simulink model "cantx_0x191"  (R2022a)
settings: configuration reference "SLDD_CFG" (kept outside this file)
values from neighbouring files (symbols this model uses):
  PLCANI_APCNTL_SET_INF_2X = 0    [cantx_0x191.sldd]
  PLCANI_APCNTL_SET_INF_4X = 1    [cantx_0x191.sldd]
  PLCANI_APCNTL_SET_INF_8X = 2    [cantx_0x191.sldd]
  PLCANI_APCNTL_SET_INF_INIT = 99    [cantx_0x191.sldd]
libraries: simulink x12
settings Model: DataDictionary=cantx_0x191.sldd  Creator=Castiel  LastModifiedBy=Castiel
settings ConfigSetRef: SourceName=SLDD_CFG

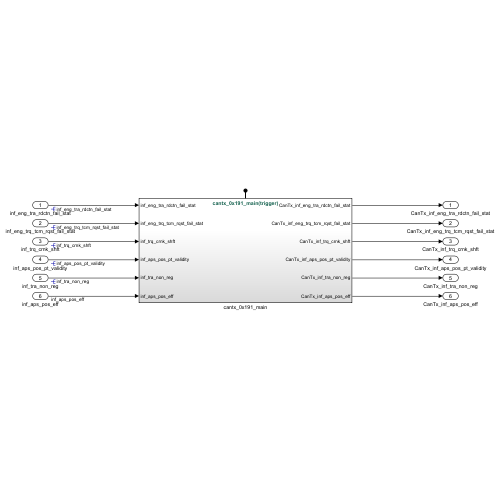
[thumbnail: Simulink's stored preview of the top-level diagram]
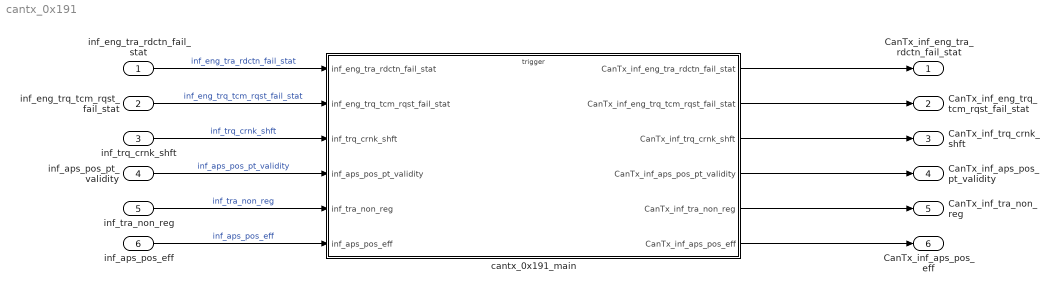
== system cantx_0x191 ==
  inf_eng_tra_rdctn_fail_stat : Inport
  inf_eng_trq_tcm_rqst_fail_stat : Inport  Port=2
  inf_trq_crnk_shft : Inport  Port=3
  inf_aps_pos_pt_validity : Inport  Port=4
  inf_tra_non_reg : Inport  Port=5
  inf_aps_pos_eff : Inport  Port=6
  cantx_0x191_main : Subsystem  TreatAsAtomicUnit=on
  CanTx_inf_eng_tra_rdctn_fail_stat : Outport  SignalName=CanTx_inf_eng_tra_rdctn_fail_stat
      settings: MustResolveToSignalObject=on
  CanTx_inf_eng_trq_tcm_rqst_fail_stat : Outport  Port=2  SignalName=CanTx_inf_eng_trq_tcm_rqst_fail_stat
      settings: MustResolveToSignalObject=on
  CanTx_inf_trq_crnk_shft : Outport  Port=3  SignalName=CanTx_inf_trq_crnk_shft
      settings: MustResolveToSignalObject=on
  CanTx_inf_aps_pos_pt_validity : Outport  Port=4  SignalName=CanTx_inf_aps_pos_pt_validity
      settings: MustResolveToSignalObject=on
  CanTx_inf_tra_non_reg : Outport  Port=5  SignalName=CanTx_inf_tra_non_reg
      settings: MustResolveToSignalObject=on
  CanTx_inf_aps_pos_eff : Outport  Port=6  SignalName=CanTx_inf_aps_pos_eff
      settings: MustResolveToSignalObject=on
  wires:
  inf_eng_tra_rdctn_fail_stat/1 -> cantx_0x191_main/1(inf_eng_tra_rdctn_fail_stat)  "inf_eng_tra_rdctn_fail_stat"
  inf_eng_trq_tcm_rqst_fail_stat/1 -> cantx_0x191_main/2(inf_eng_trq_tcm_rqst_fail_stat)  "inf_eng_trq_tcm_rqst_fail_stat"
  inf_trq_crnk_shft/1 -> cantx_0x191_main/3(inf_trq_crnk_shft)  "inf_trq_crnk_shft"
  inf_aps_pos_pt_validity/1 -> cantx_0x191_main/4(inf_aps_pos_pt_validity)  "inf_aps_pos_pt_validity"
  inf_tra_non_reg/1 -> cantx_0x191_main/5(inf_tra_non_reg)  "inf_tra_non_reg"
  inf_aps_pos_eff/1 -> cantx_0x191_main/6(inf_aps_pos_eff)  "inf_aps_pos_eff"
  cantx_0x191_main/1(CanTx_inf_eng_tra_rdctn_fail_stat) -> CanTx_inf_eng_tra_rdctn_fail_stat/1
  cantx_0x191_main/2(CanTx_inf_eng_trq_tcm_rqst_fail_stat) -> CanTx_inf_eng_trq_tcm_rqst_fail_stat/1
  cantx_0x191_main/3(CanTx_inf_trq_crnk_shft) -> CanTx_inf_trq_crnk_shft/1
  cantx_0x191_main/4(CanTx_inf_aps_pos_pt_validity) -> CanTx_inf_aps_pos_pt_validity/1
  cantx_0x191_main/5(CanTx_inf_tra_non_reg) -> CanTx_inf_tra_non_reg/1
  cantx_0x191_main/6(CanTx_inf_aps_pos_eff) -> CanTx_inf_aps_pos_eff/1

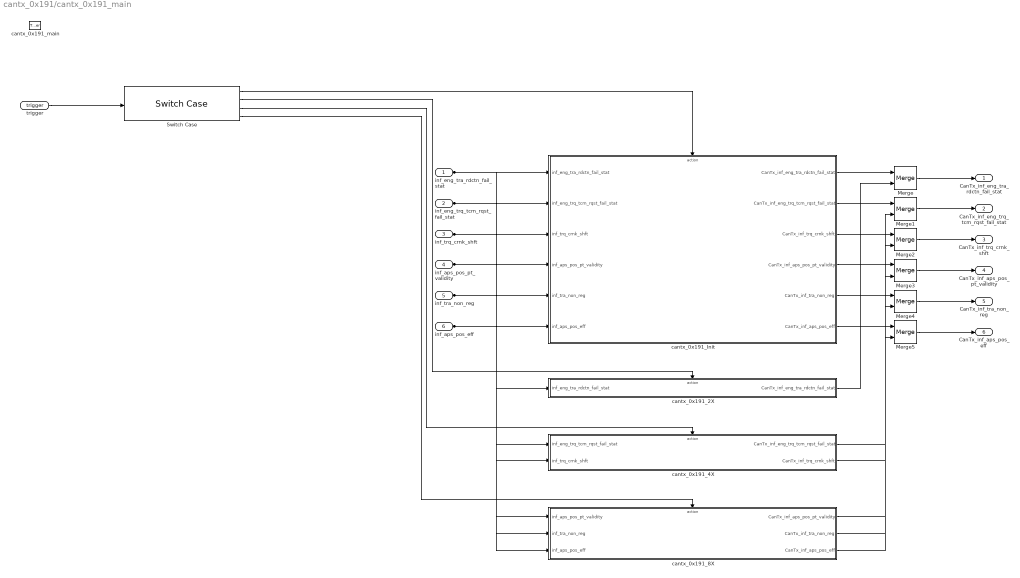
== system cantx_0x191/cantx_0x191_main ==
  inf_eng_tra_rdctn_fail_stat : Inport
  inf_eng_trq_tcm_rqst_fail_stat : Inport  Port=2
  inf_trq_crnk_shft : Inport  Port=3
  inf_aps_pos_pt_validity : Inport  Port=4
  inf_tra_non_reg : Inport  Port=5
  inf_aps_pos_eff : Inport  Port=6
  cantx_0x191_main : TriggerPort  TriggerType=function-call  IsSimulinkFunction=on  FunctionName=cantx_0x191_main  FunctionVisibility=scoped  VariantControl=(inherit)
  Merge{,1..5} (6 alike) : Merge
  Switch Case : SwitchCase  CaseConditions={PLCANI_APCNTL_SET_INF_TYPE.PLCANI_APCNTL_SET_INF_INIT,PLCANI_APCNTL_SET_INF_TYPE.PLCANI_APCNTL_SET_INF_2X,PLCANI_APCNTL_SET_INF_TYPE.PLCANI_APCNTL_SET_INF_4X,PLCANI_APCNTL_SET_INF_TYPE.PLCANI_APCNTL_SET_INF_8X}  ShowDefaultCase=off
  cantx_0x191_2X : Subsystem  TreatAsAtomicUnit=on
      settings: RTWFcnNameOpts=Use subsystem name
  cantx_0x191_4X : Subsystem  TreatAsAtomicUnit=on
      settings: RTWFcnNameOpts=Use subsystem name
  cantx_0x191_8X : Subsystem  TreatAsAtomicUnit=on
      settings: RTWFcnNameOpts=Use subsystem name
  cantx_0x191_Init : Subsystem  TreatAsAtomicUnit=on
      settings: RTWFcnNameOpts=Use subsystem name
  trigger : ArgIn  DisableCoverage=on  OutDataTypeStr=Enum: PLCANI_APCNTL_SET_INF_TYPE  ArgumentName=trigger
  CanTx_inf_eng_tra_rdctn_fail_stat : Outport
  CanTx_inf_eng_trq_tcm_rqst_fail_stat : Outport  Port=2
  CanTx_inf_trq_crnk_shft : Outport  Port=3
  CanTx_inf_aps_pos_pt_validity : Outport  Port=4
  CanTx_inf_tra_non_reg : Outport  Port=5
  CanTx_inf_aps_pos_eff : Outport  Port=6
  wires:
  trigger/1 -> Switch Case/1
  Switch Case/1 -> cantx_0x191_Init/Action
  inf_eng_tra_rdctn_fail_stat/1 -> cantx_0x191_Init/1(inf_eng_tra_rdctn_fail_stat), cantx_0x191_2X/1(inf_eng_tra_rdctn_fail_stat)
  inf_eng_trq_tcm_rqst_fail_stat/1 -> cantx_0x191_Init/2(inf_eng_trq_tcm_rqst_fail_stat), cantx_0x191_4X/1(inf_eng_trq_tcm_rqst_fail_stat)
  inf_trq_crnk_shft/1 -> cantx_0x191_Init/3(inf_trq_crnk_shft), cantx_0x191_4X/2(inf_trq_crnk_shft)
  inf_aps_pos_pt_validity/1 -> cantx_0x191_Init/4(inf_aps_pos_pt_validity), cantx_0x191_8X/1(inf_aps_pos_pt_validity)
  inf_tra_non_reg/1 -> cantx_0x191_Init/5(inf_tra_non_reg), cantx_0x191_8X/2(inf_tra_non_reg)
  inf_aps_pos_eff/1 -> cantx_0x191_Init/6(inf_aps_pos_eff), cantx_0x191_8X/3(inf_aps_pos_eff)
  Switch Case/2 -> cantx_0x191_2X/Action
  cantx_0x191_Init/1(CanTx_inf_eng_tra_rdctn_fail_stat) -> Merge/1
  cantx_0x191_2X/1(CanTx_inf_eng_tra_rdctn_fail_stat) -> Merge/2
  Merge/1 -> CanTx_inf_eng_tra_rdctn_fail_stat/1
  Switch Case/3 -> cantx_0x191_4X/Action
  cantx_0x191_Init/2(CanTx_inf_eng_trq_tcm_rqst_fail_stat) -> Merge1/1
  cantx_0x191_4X/1(CanTx_inf_eng_trq_tcm_rqst_fail_stat) -> Merge1/2
  Merge1/1 -> CanTx_inf_eng_trq_tcm_rqst_fail_stat/1
  cantx_0x191_Init/3(CanTx_inf_trq_crnk_shft) -> Merge2/1
  cantx_0x191_4X/2(CanTx_inf_trq_crnk_shft) -> Merge2/2
  Merge2/1 -> CanTx_inf_trq_crnk_shft/1
  Switch Case/4 -> cantx_0x191_8X/Action
  cantx_0x191_Init/4(CanTx_inf_aps_pos_pt_validity) -> Merge3/1
  cantx_0x191_8X/1(CanTx_inf_aps_pos_pt_validity) -> Merge3/2
  Merge3/1 -> CanTx_inf_aps_pos_pt_validity/1
  cantx_0x191_Init/5(CanTx_inf_tra_non_reg) -> Merge4/1
  cantx_0x191_8X/2(CanTx_inf_tra_non_reg) -> Merge4/2
  Merge4/1 -> CanTx_inf_tra_non_reg/1
  cantx_0x191_Init/6(CanTx_inf_aps_pos_eff) -> Merge5/1
  cantx_0x191_8X/3(CanTx_inf_aps_pos_eff) -> Merge5/2
  Merge5/1 -> CanTx_inf_aps_pos_eff/1

== system cantx_0x191/cantx_0x191_main/cantx_0x191_2X ==
  inf_eng_tra_rdctn_fail_stat : Inport
  Action Port : ActionPort  ActionPortLabel=case [ PLCANI_APCNTL_SET_INF_2X ]:
  sig_inf_eng_tra_rdctn_fail_stat : Subsystem  TreatAsAtomicUnit=on
      settings: RTWFcnNameOpts=Use subsystem name
  CanTx_inf_eng_tra_rdctn_fail_stat : Outport
  wires:
  inf_eng_tra_rdctn_fail_stat/1 -> sig_inf_eng_tra_rdctn_fail_stat/1(inf_eng_tra_rdctn_fail_stat)
  sig_inf_eng_tra_rdctn_fail_stat/1(CanTx_inf_eng_tra_rdctn_fail_stat) -> CanTx_inf_eng_tra_rdctn_fail_stat/1

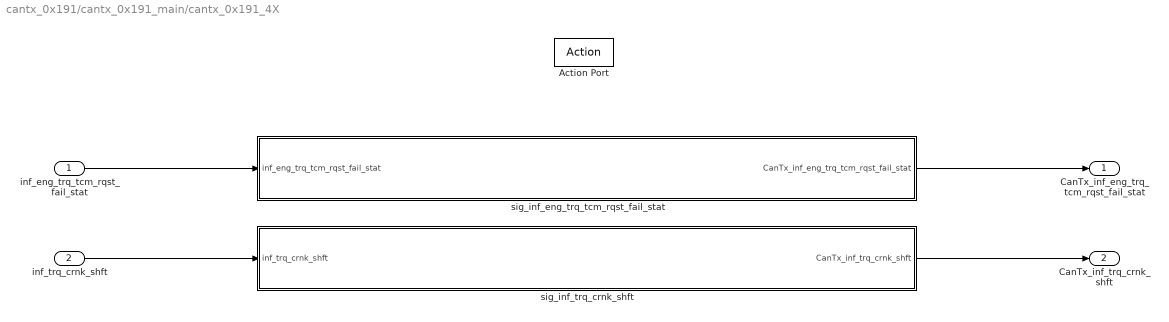
== system cantx_0x191/cantx_0x191_main/cantx_0x191_4X ==
  inf_eng_trq_tcm_rqst_fail_stat : Inport
  inf_trq_crnk_shft : Inport  Port=2
  Action Port : ActionPort  ActionPortLabel=case [ PLCANI_APCNTL_SET_INF_4X ]:
  sig_inf_eng_trq_tcm_rqst_fail_stat : Subsystem  TreatAsAtomicUnit=on
      settings: RTWFcnNameOpts=Use subsystem name
  sig_inf_trq_crnk_shft : Subsystem  TreatAsAtomicUnit=on
      settings: RTWFcnNameOpts=Use subsystem name
  CanTx_inf_eng_trq_tcm_rqst_fail_stat : Outport
  CanTx_inf_trq_crnk_shft : Outport  Port=2
  wires:
  inf_eng_trq_tcm_rqst_fail_stat/1 -> sig_inf_eng_trq_tcm_rqst_fail_stat/1(inf_eng_trq_tcm_rqst_fail_stat)
  sig_inf_eng_trq_tcm_rqst_fail_stat/1(CanTx_inf_eng_trq_tcm_rqst_fail_stat) -> CanTx_inf_eng_trq_tcm_rqst_fail_stat/1
  inf_trq_crnk_shft/1 -> sig_inf_trq_crnk_shft/1(inf_trq_crnk_shft)
  sig_inf_trq_crnk_shft/1(CanTx_inf_trq_crnk_shft) -> CanTx_inf_trq_crnk_shft/1

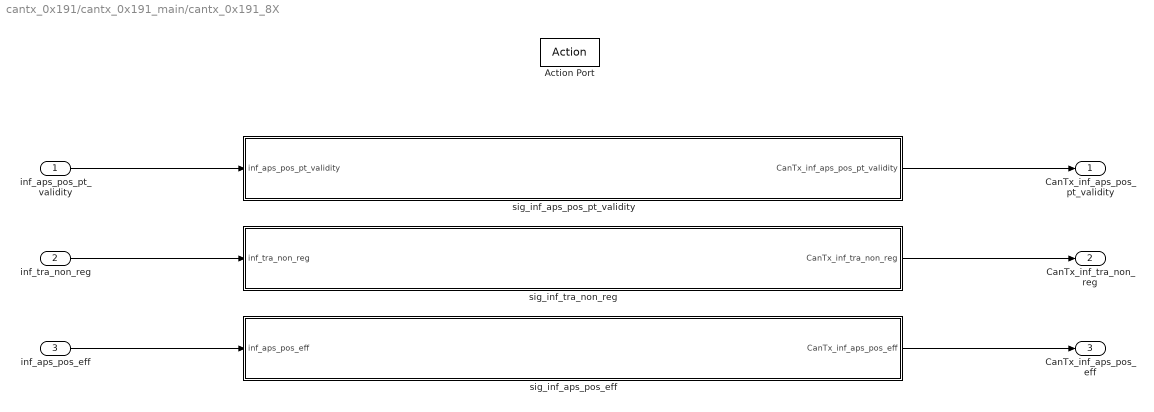
== system cantx_0x191/cantx_0x191_main/cantx_0x191_8X ==
  inf_aps_pos_pt_validity : Inport
  inf_tra_non_reg : Inport  Port=2
  inf_aps_pos_eff : Inport  Port=3
  Action Port : ActionPort  ActionPortLabel=case [ PLCANI_APCNTL_SET_INF_8X ]:
  sig_inf_aps_pos_eff : Subsystem  TreatAsAtomicUnit=on
      settings: RTWFcnNameOpts=Use subsystem name
  sig_inf_aps_pos_pt_validity : Subsystem  TreatAsAtomicUnit=on
      settings: RTWFcnNameOpts=Use subsystem name
  sig_inf_tra_non_reg : Subsystem  TreatAsAtomicUnit=on
      settings: RTWFcnNameOpts=Use subsystem name
  CanTx_inf_aps_pos_pt_validity : Outport
  CanTx_inf_tra_non_reg : Outport  Port=2
  CanTx_inf_aps_pos_eff : Outport  Port=3
  wires:
  inf_aps_pos_pt_validity/1 -> sig_inf_aps_pos_pt_validity/1(inf_aps_pos_pt_validity)
  sig_inf_aps_pos_pt_validity/1(CanTx_inf_aps_pos_pt_validity) -> CanTx_inf_aps_pos_pt_validity/1
  inf_tra_non_reg/1 -> sig_inf_tra_non_reg/1(inf_tra_non_reg)
  sig_inf_tra_non_reg/1(CanTx_inf_tra_non_reg) -> CanTx_inf_tra_non_reg/1
  inf_aps_pos_eff/1 -> sig_inf_aps_pos_eff/1(inf_aps_pos_eff)
  sig_inf_aps_pos_eff/1(CanTx_inf_aps_pos_eff) -> CanTx_inf_aps_pos_eff/1

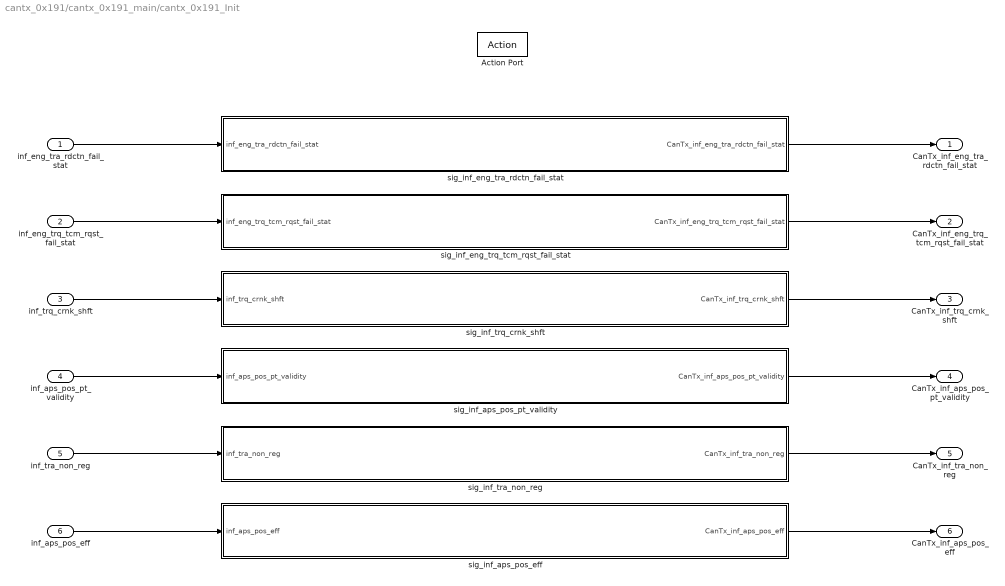
== system cantx_0x191/cantx_0x191_main/cantx_0x191_Init ==
  inf_eng_tra_rdctn_fail_stat : Inport
  inf_eng_trq_tcm_rqst_fail_stat : Inport  Port=2
  inf_trq_crnk_shft : Inport  Port=3
  inf_aps_pos_pt_validity : Inport  Port=4
  inf_tra_non_reg : Inport  Port=5
  inf_aps_pos_eff : Inport  Port=6
  Action Port : ActionPort  ActionPortLabel=case [ PLCANI_APCNTL_SET_INF_INIT ]:
  sig_inf_aps_pos_eff : Subsystem  TreatAsAtomicUnit=on
      settings: RTWFcnNameOpts=Use subsystem name
  sig_inf_aps_pos_pt_validity : Subsystem  TreatAsAtomicUnit=on
      settings: RTWFcnNameOpts=Use subsystem name
  sig_inf_eng_tra_rdctn_fail_stat : Subsystem  TreatAsAtomicUnit=on
      settings: RTWFcnNameOpts=Use subsystem name
  sig_inf_eng_trq_tcm_rqst_fail_stat : Subsystem  TreatAsAtomicUnit=on
      settings: RTWFcnNameOpts=Use subsystem name
  sig_inf_tra_non_reg : Subsystem  TreatAsAtomicUnit=on
      settings: RTWFcnNameOpts=Use subsystem name
  sig_inf_trq_crnk_shft : Subsystem  TreatAsAtomicUnit=on
      settings: RTWFcnNameOpts=Use subsystem name
  CanTx_inf_eng_tra_rdctn_fail_stat : Outport
  CanTx_inf_eng_trq_tcm_rqst_fail_stat : Outport  Port=2
  CanTx_inf_trq_crnk_shft : Outport  Port=3
  CanTx_inf_aps_pos_pt_validity : Outport  Port=4
  CanTx_inf_tra_non_reg : Outport  Port=5
  CanTx_inf_aps_pos_eff : Outport  Port=6
  wires:
  inf_eng_tra_rdctn_fail_stat/1 -> sig_inf_eng_tra_rdctn_fail_stat/1(inf_eng_tra_rdctn_fail_stat)
  sig_inf_eng_tra_rdctn_fail_stat/1(CanTx_inf_eng_tra_rdctn_fail_stat) -> CanTx_inf_eng_tra_rdctn_fail_stat/1
  inf_eng_trq_tcm_rqst_fail_stat/1 -> sig_inf_eng_trq_tcm_rqst_fail_stat/1(inf_eng_trq_tcm_rqst_fail_stat)
  sig_inf_eng_trq_tcm_rqst_fail_stat/1(CanTx_inf_eng_trq_tcm_rqst_fail_stat) -> CanTx_inf_eng_trq_tcm_rqst_fail_stat/1
  inf_trq_crnk_shft/1 -> sig_inf_trq_crnk_shft/1(inf_trq_crnk_shft)
  sig_inf_trq_crnk_shft/1(CanTx_inf_trq_crnk_shft) -> CanTx_inf_trq_crnk_shft/1
  inf_aps_pos_pt_validity/1 -> sig_inf_aps_pos_pt_validity/1(inf_aps_pos_pt_validity)
  sig_inf_aps_pos_pt_validity/1(CanTx_inf_aps_pos_pt_validity) -> CanTx_inf_aps_pos_pt_validity/1
  inf_tra_non_reg/1 -> sig_inf_tra_non_reg/1(inf_tra_non_reg)
  sig_inf_tra_non_reg/1(CanTx_inf_tra_non_reg) -> CanTx_inf_tra_non_reg/1
  inf_aps_pos_eff/1 -> sig_inf_aps_pos_eff/1(inf_aps_pos_eff)
  sig_inf_aps_pos_eff/1(CanTx_inf_aps_pos_eff) -> CanTx_inf_aps_pos_eff/1

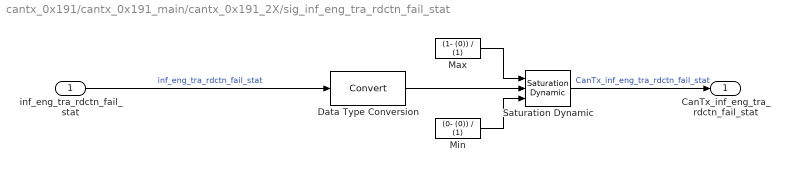
== system cantx_0x191/cantx_0x191_main/cantx_0x191_2X/sig_inf_eng_tra_rdctn_fail_stat ==
  inf_eng_tra_rdctn_fail_stat : Inport
  Data Type Conversion : DataTypeConversion  SaturateOnIntegerOverflow=off  RndMeth=Floor
  Max : Constant  Value=(1- (0)) / (1)  OutDataTypeStr=Inherit: Inherit via back propagation
  Min : Constant  Value=(0- (0)) / (1)  OutDataTypeStr=Inherit: Inherit via back propagation
  Saturation Dynamic : simulink/Discontinuities/Saturation Dynamic  OutMin=[]  OutMax=[]  OutDataTypeStr=Inherit: Same as second input  OutDataType=fixdt(1, 16)  OutScaling=2^-10  DoSatur=off
  CanTx_inf_eng_tra_rdctn_fail_stat : Outport
  wires:
  Saturation Dynamic/1 -> CanTx_inf_eng_tra_rdctn_fail_stat/1  "CanTx_inf_eng_tra_rdctn_fail_stat"
  Data Type Conversion/1 -> Saturation Dynamic/2
  inf_eng_tra_rdctn_fail_stat/1 -> Data Type Conversion/1  "inf_eng_tra_rdctn_fail_stat"
  Min/1 -> Saturation Dynamic/3
  Max/1 -> Saturation Dynamic/1

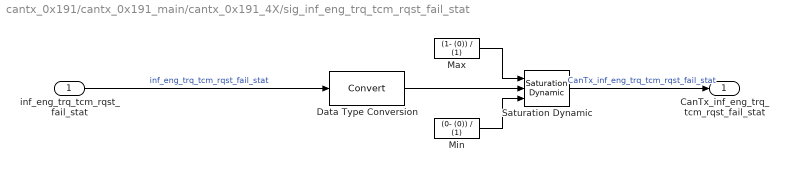
== system cantx_0x191/cantx_0x191_main/cantx_0x191_4X/sig_inf_eng_trq_tcm_rqst_fail_stat ==
  inf_eng_trq_tcm_rqst_fail_stat : Inport
  Data Type Conversion : DataTypeConversion  SaturateOnIntegerOverflow=off  RndMeth=Floor
  Max : Constant  Value=(1- (0)) / (1)  OutDataTypeStr=Inherit: Inherit via back propagation
  Min : Constant  Value=(0- (0)) / (1)  OutDataTypeStr=Inherit: Inherit via back propagation
  Saturation Dynamic : simulink/Discontinuities/Saturation Dynamic  OutMin=[]  OutMax=[]  OutDataTypeStr=Inherit: Same as second input  OutDataType=fixdt(1, 16)  OutScaling=2^-10  DoSatur=off
  CanTx_inf_eng_trq_tcm_rqst_fail_stat : Outport
  wires:
  Saturation Dynamic/1 -> CanTx_inf_eng_trq_tcm_rqst_fail_stat/1  "CanTx_inf_eng_trq_tcm_rqst_fail_stat"
  Data Type Conversion/1 -> Saturation Dynamic/2
  inf_eng_trq_tcm_rqst_fail_stat/1 -> Data Type Conversion/1  "inf_eng_trq_tcm_rqst_fail_stat"
  Min/1 -> Saturation Dynamic/3
  Max/1 -> Saturation Dynamic/1

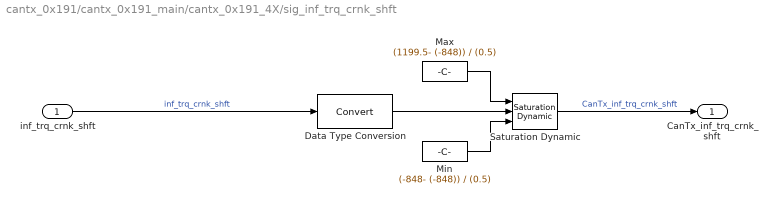
== system cantx_0x191/cantx_0x191_main/cantx_0x191_4X/sig_inf_trq_crnk_shft ==
  inf_trq_crnk_shft : Inport
  Data Type Conversion : DataTypeConversion  SaturateOnIntegerOverflow=off  RndMeth=Floor
  Max : Constant  Value=(1199.5- (-848)) / (0.5)  OutDataTypeStr=Inherit: Inherit via back propagation
  Min : Constant  Value=(-848- (-848)) / (0.5)  OutDataTypeStr=Inherit: Inherit via back propagation
  Saturation Dynamic : simulink/Discontinuities/Saturation Dynamic  OutMin=[]  OutMax=[]  OutDataTypeStr=Inherit: Same as second input  OutDataType=fixdt(1, 16)  OutScaling=2^-10  DoSatur=off
  CanTx_inf_trq_crnk_shft : Outport
  wires:
  Saturation Dynamic/1 -> CanTx_inf_trq_crnk_shft/1  "CanTx_inf_trq_crnk_shft"
  Data Type Conversion/1 -> Saturation Dynamic/2
  inf_trq_crnk_shft/1 -> Data Type Conversion/1  "inf_trq_crnk_shft"
  Min/1 -> Saturation Dynamic/3
  Max/1 -> Saturation Dynamic/1

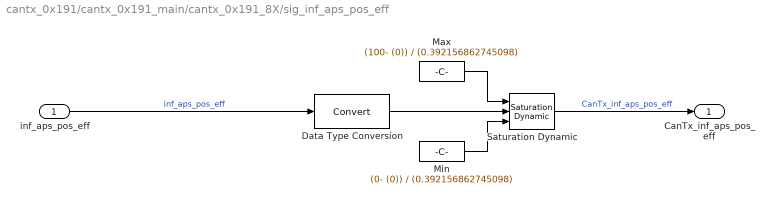
== system cantx_0x191/cantx_0x191_main/cantx_0x191_8X/sig_inf_aps_pos_eff ==
  inf_aps_pos_eff : Inport
  Data Type Conversion : DataTypeConversion  SaturateOnIntegerOverflow=off  RndMeth=Floor
  Max : Constant  Value=(100- (0)) / (0.392156862745098)  OutDataTypeStr=Inherit: Inherit via back propagation
  Min : Constant  Value=(0- (0)) / (0.392156862745098)  OutDataTypeStr=Inherit: Inherit via back propagation
  Saturation Dynamic : simulink/Discontinuities/Saturation Dynamic  OutMin=[]  OutMax=[]  OutDataTypeStr=Inherit: Same as second input  OutDataType=fixdt(1, 16)  OutScaling=2^-10  DoSatur=off
  CanTx_inf_aps_pos_eff : Outport
  wires:
  Saturation Dynamic/1 -> CanTx_inf_aps_pos_eff/1  "CanTx_inf_aps_pos_eff"
  Data Type Conversion/1 -> Saturation Dynamic/2
  inf_aps_pos_eff/1 -> Data Type Conversion/1  "inf_aps_pos_eff"
  Min/1 -> Saturation Dynamic/3
  Max/1 -> Saturation Dynamic/1

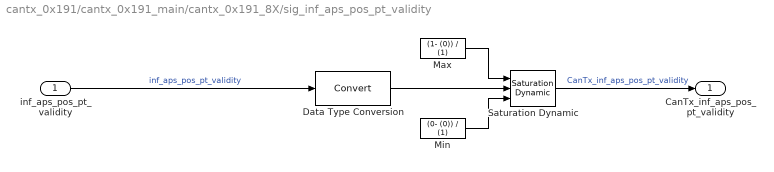
== system cantx_0x191/cantx_0x191_main/cantx_0x191_8X/sig_inf_aps_pos_pt_validity ==
  inf_aps_pos_pt_validity : Inport
  Data Type Conversion : DataTypeConversion  SaturateOnIntegerOverflow=off  RndMeth=Floor
  Max : Constant  Value=(1- (0)) / (1)  OutDataTypeStr=Inherit: Inherit via back propagation
  Min : Constant  Value=(0- (0)) / (1)  OutDataTypeStr=Inherit: Inherit via back propagation
  Saturation Dynamic : simulink/Discontinuities/Saturation Dynamic  OutMin=[]  OutMax=[]  OutDataTypeStr=Inherit: Same as second input  OutDataType=fixdt(1, 16)  OutScaling=2^-10  DoSatur=off
  CanTx_inf_aps_pos_pt_validity : Outport
  wires:
  Saturation Dynamic/1 -> CanTx_inf_aps_pos_pt_validity/1  "CanTx_inf_aps_pos_pt_validity"
  Data Type Conversion/1 -> Saturation Dynamic/2
  inf_aps_pos_pt_validity/1 -> Data Type Conversion/1  "inf_aps_pos_pt_validity"
  Min/1 -> Saturation Dynamic/3
  Max/1 -> Saturation Dynamic/1

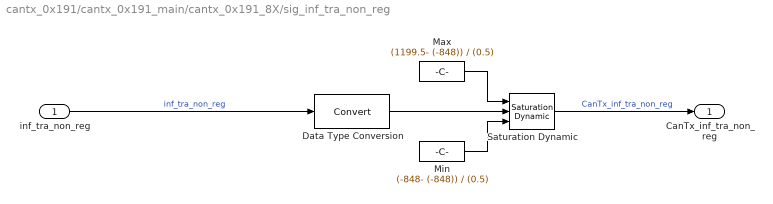
== system cantx_0x191/cantx_0x191_main/cantx_0x191_8X/sig_inf_tra_non_reg ==
  inf_tra_non_reg : Inport
  Data Type Conversion : DataTypeConversion  SaturateOnIntegerOverflow=off  RndMeth=Floor
  Max : Constant  Value=(1199.5- (-848)) / (0.5)  OutDataTypeStr=Inherit: Inherit via back propagation
  Min : Constant  Value=(-848- (-848)) / (0.5)  OutDataTypeStr=Inherit: Inherit via back propagation
  Saturation Dynamic : simulink/Discontinuities/Saturation Dynamic  OutMin=[]  OutMax=[]  OutDataTypeStr=Inherit: Same as second input  OutDataType=fixdt(1, 16)  OutScaling=2^-10  DoSatur=off
  CanTx_inf_tra_non_reg : Outport
  wires:
  Saturation Dynamic/1 -> CanTx_inf_tra_non_reg/1  "CanTx_inf_tra_non_reg"
  Data Type Conversion/1 -> Saturation Dynamic/2
  inf_tra_non_reg/1 -> Data Type Conversion/1  "inf_tra_non_reg"
  Min/1 -> Saturation Dynamic/3
  Max/1 -> Saturation Dynamic/1

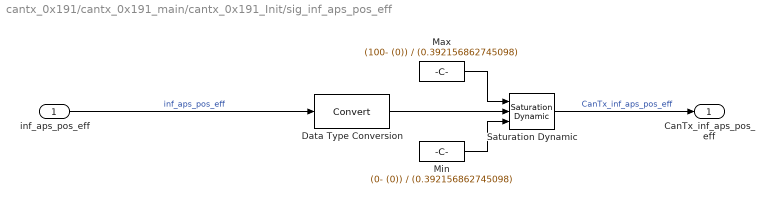
== system cantx_0x191/cantx_0x191_main/cantx_0x191_Init/sig_inf_aps_pos_eff ==
  inf_aps_pos_eff : Inport
  Data Type Conversion : DataTypeConversion  SaturateOnIntegerOverflow=off  RndMeth=Floor
  Max : Constant  Value=(100- (0)) / (0.392156862745098)  OutDataTypeStr=Inherit: Inherit via back propagation
  Min : Constant  Value=(0- (0)) / (0.392156862745098)  OutDataTypeStr=Inherit: Inherit via back propagation
  Saturation Dynamic : simulink/Discontinuities/Saturation Dynamic  OutMin=[]  OutMax=[]  OutDataTypeStr=Inherit: Same as second input  OutDataType=fixdt(1, 16)  OutScaling=2^-10  DoSatur=off
  CanTx_inf_aps_pos_eff : Outport
  wires:
  Saturation Dynamic/1 -> CanTx_inf_aps_pos_eff/1  "CanTx_inf_aps_pos_eff"
  Data Type Conversion/1 -> Saturation Dynamic/2
  inf_aps_pos_eff/1 -> Data Type Conversion/1  "inf_aps_pos_eff"
  Min/1 -> Saturation Dynamic/3
  Max/1 -> Saturation Dynamic/1

== system cantx_0x191/cantx_0x191_main/cantx_0x191_Init/sig_inf_aps_pos_pt_validity ==
  inf_aps_pos_pt_validity : Inport
  Data Type Conversion : DataTypeConversion  SaturateOnIntegerOverflow=off  RndMeth=Floor
  Max : Constant  Value=(1- (0)) / (1)  OutDataTypeStr=Inherit: Inherit via back propagation
  Min : Constant  Value=(0- (0)) / (1)  OutDataTypeStr=Inherit: Inherit via back propagation
  Saturation Dynamic : simulink/Discontinuities/Saturation Dynamic  OutMin=[]  OutMax=[]  OutDataTypeStr=Inherit: Same as second input  OutDataType=fixdt(1, 16)  OutScaling=2^-10  DoSatur=off
  CanTx_inf_aps_pos_pt_validity : Outport
  wires:
  Saturation Dynamic/1 -> CanTx_inf_aps_pos_pt_validity/1  "CanTx_inf_aps_pos_pt_validity"
  Data Type Conversion/1 -> Saturation Dynamic/2
  inf_aps_pos_pt_validity/1 -> Data Type Conversion/1  "inf_aps_pos_pt_validity"
  Min/1 -> Saturation Dynamic/3
  Max/1 -> Saturation Dynamic/1

== system cantx_0x191/cantx_0x191_main/cantx_0x191_Init/sig_inf_eng_tra_rdctn_fail_stat ==
  inf_eng_tra_rdctn_fail_stat : Inport
  Data Type Conversion : DataTypeConversion  SaturateOnIntegerOverflow=off  RndMeth=Floor
  Max : Constant  Value=(1- (0)) / (1)  OutDataTypeStr=Inherit: Inherit via back propagation
  Min : Constant  Value=(0- (0)) / (1)  OutDataTypeStr=Inherit: Inherit via back propagation
  Saturation Dynamic : simulink/Discontinuities/Saturation Dynamic  OutMin=[]  OutMax=[]  OutDataTypeStr=Inherit: Same as second input  OutDataType=fixdt(1, 16)  OutScaling=2^-10  DoSatur=off
  CanTx_inf_eng_tra_rdctn_fail_stat : Outport
  wires:
  Saturation Dynamic/1 -> CanTx_inf_eng_tra_rdctn_fail_stat/1  "CanTx_inf_eng_tra_rdctn_fail_stat"
  Data Type Conversion/1 -> Saturation Dynamic/2
  inf_eng_tra_rdctn_fail_stat/1 -> Data Type Conversion/1  "inf_eng_tra_rdctn_fail_stat"
  Min/1 -> Saturation Dynamic/3
  Max/1 -> Saturation Dynamic/1

== system cantx_0x191/cantx_0x191_main/cantx_0x191_Init/sig_inf_eng_trq_tcm_rqst_fail_stat ==
  inf_eng_trq_tcm_rqst_fail_stat : Inport
  Data Type Conversion : DataTypeConversion  SaturateOnIntegerOverflow=off  RndMeth=Floor
  Max : Constant  Value=(1- (0)) / (1)  OutDataTypeStr=Inherit: Inherit via back propagation
  Min : Constant  Value=(0- (0)) / (1)  OutDataTypeStr=Inherit: Inherit via back propagation
  Saturation Dynamic : simulink/Discontinuities/Saturation Dynamic  OutMin=[]  OutMax=[]  OutDataTypeStr=Inherit: Same as second input  OutDataType=fixdt(1, 16)  OutScaling=2^-10  DoSatur=off
  CanTx_inf_eng_trq_tcm_rqst_fail_stat : Outport
  wires:
  Saturation Dynamic/1 -> CanTx_inf_eng_trq_tcm_rqst_fail_stat/1  "CanTx_inf_eng_trq_tcm_rqst_fail_stat"
  Data Type Conversion/1 -> Saturation Dynamic/2
  inf_eng_trq_tcm_rqst_fail_stat/1 -> Data Type Conversion/1  "inf_eng_trq_tcm_rqst_fail_stat"
  Min/1 -> Saturation Dynamic/3
  Max/1 -> Saturation Dynamic/1

== system cantx_0x191/cantx_0x191_main/cantx_0x191_Init/sig_inf_tra_non_reg ==
  inf_tra_non_reg : Inport
  Data Type Conversion : DataTypeConversion  SaturateOnIntegerOverflow=off  RndMeth=Floor
  Max : Constant  Value=(1199.5- (-848)) / (0.5)  OutDataTypeStr=Inherit: Inherit via back propagation
  Min : Constant  Value=(-848- (-848)) / (0.5)  OutDataTypeStr=Inherit: Inherit via back propagation
  Saturation Dynamic : simulink/Discontinuities/Saturation Dynamic  OutMin=[]  OutMax=[]  OutDataTypeStr=Inherit: Same as second input  OutDataType=fixdt(1, 16)  OutScaling=2^-10  DoSatur=off
  CanTx_inf_tra_non_reg : Outport
  wires:
  Saturation Dynamic/1 -> CanTx_inf_tra_non_reg/1  "CanTx_inf_tra_non_reg"
  Data Type Conversion/1 -> Saturation Dynamic/2
  inf_tra_non_reg/1 -> Data Type Conversion/1  "inf_tra_non_reg"
  Min/1 -> Saturation Dynamic/3
  Max/1 -> Saturation Dynamic/1

== system cantx_0x191/cantx_0x191_main/cantx_0x191_Init/sig_inf_trq_crnk_shft ==
  inf_trq_crnk_shft : Inport
  Data Type Conversion : DataTypeConversion  SaturateOnIntegerOverflow=off  RndMeth=Floor
  Max : Constant  Value=(1199.5- (-848)) / (0.5)  OutDataTypeStr=Inherit: Inherit via back propagation
  Min : Constant  Value=(-848- (-848)) / (0.5)  OutDataTypeStr=Inherit: Inherit via back propagation
  Saturation Dynamic : simulink/Discontinuities/Saturation Dynamic  OutMin=[]  OutMax=[]  OutDataTypeStr=Inherit: Same as second input  OutDataType=fixdt(1, 16)  OutScaling=2^-10  DoSatur=off
  CanTx_inf_trq_crnk_shft : Outport
  wires:
  Saturation Dynamic/1 -> CanTx_inf_trq_crnk_shft/1  "CanTx_inf_trq_crnk_shft"
  Data Type Conversion/1 -> Saturation Dynamic/2
  inf_trq_crnk_shft/1 -> Data Type Conversion/1  "inf_trq_crnk_shft"
  Min/1 -> Saturation Dynamic/3
  Max/1 -> Saturation Dynamic/1
